simulink model "udp_send"  (R2015a)
settings: Solver=FixedStepDiscrete  StartTime=0.0  StopTime=inf  FixedStep=0.01  RelTol=1e-3
libraries: dspnetwork x2, etargetslib x1, xpcutilitieslib x1
settings Model: Creator=Centauro  LastModifiedBy=Centauro
settings SolverCC: AutoInsertRateTranBlk=on

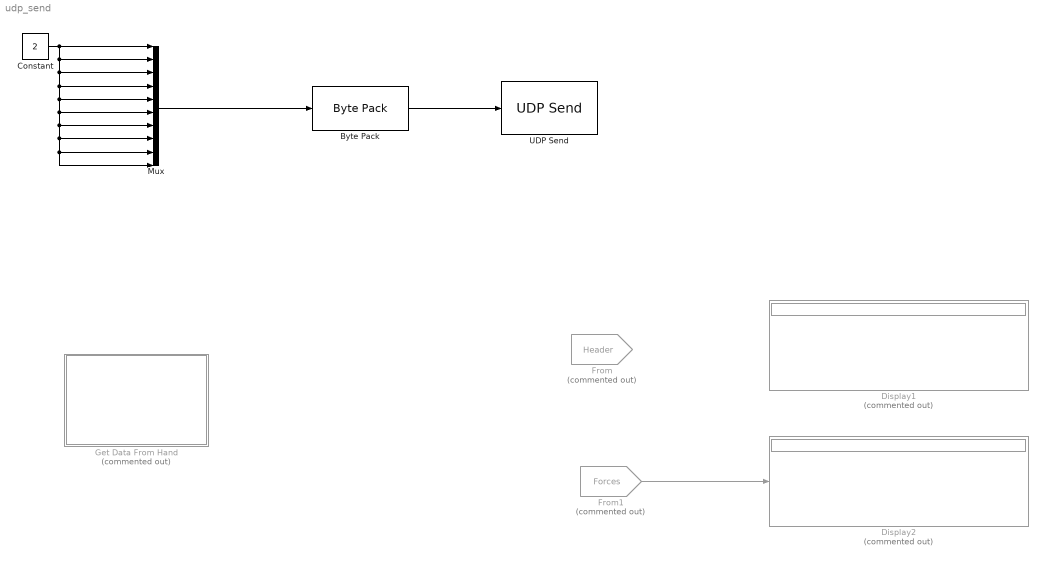
== system udp_send ==
  Byte Pack : etargetslib/Byte Pack  datatypes={'single'}  byteAlign=1
  Constant : Constant  Value=2  OutDataTypeStr=single
  Display1 : Display  Commented=on
  Display2 : Display  Commented=on
  From : From  Commented=on  GotoTag=Header  TagVisibility=global
  From1 : From  Commented=on  GotoTag=Forces  TagVisibility=global
  Get Data From Hand : Subsystem  Commented=on
  Mux : Mux  Inputs=10
  UDP Send : dspnetwork/UDP Send  remoteURL='10.100.39.22'  remotePort=12005  localURL='0.0.0.0'  localPortSource=Automatically determine  localPort=-1  sampletime=-1  blockPlatform=HOST  separateLengthPort=0
  wires:
  Byte Pack/1 -> UDP Send/1
  Mux/1 -> Byte Pack/1
  Constant/1 -> Mux/2, Mux/3, Mux/4, Mux/5, Mux/6, Mux/7, Mux/8, Mux/9, Mux/10, Mux/1
  From1/1 -> Display2/1

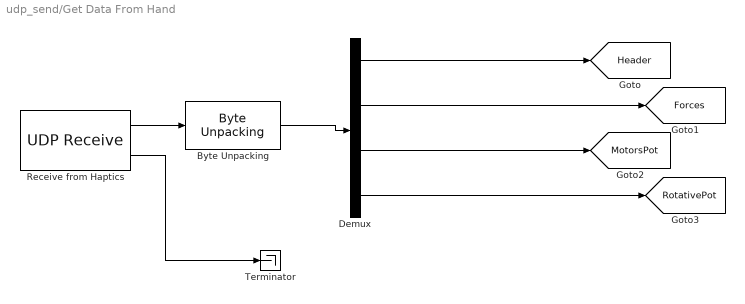
== system udp_send/Get Data From Hand ==
  "Byte Unpacking " : xpcutilitieslib/Byte Unpacking   MaskUnpackedDataTypes={'single'}  MaskUnpackedDataSizes={[17]}  MaskAlignment=1
  Demux : Demux  Outputs=[2, 5, 5, 5]
  Receive from Haptics : dspnetwork/UDP Receive  localURL='0.0.0.0'  localPort=15001  remoteURL='10.100.39.144'  remotePort=-1  recvBufferSize=8192  dims=17*4  signalDatatype=uint8  isVarSize=off  showBlockingTime=on  blockingTime=inf  sampletime=0.01  blockPlatform=HOST
  Terminator : Terminator
  tag scope: Forces=global, Header=global, MotorsPot=global, RotativePot=global
  wires:
  Demux/3 -> [MotorsPot]
  Demux/1 -> [Header]
  Demux/4 -> [RotativePot]
  Demux/2 -> [Forces]
  "Byte Unpacking "/1 -> Demux/1
  Receive from Haptics/1 -> "Byte Unpacking "/1
  Receive from Haptics/2 -> Terminator/1
